simulink model "flexible_joint_v01"  (R2023b)
settings: Solver=FixedStepAuto  StartTime=0.0  StopTime=30  FixedStep=0.001  RelTol=1e-3
settings Model: Creator=GreenTeam  LastModifiedBy=GreenTeam

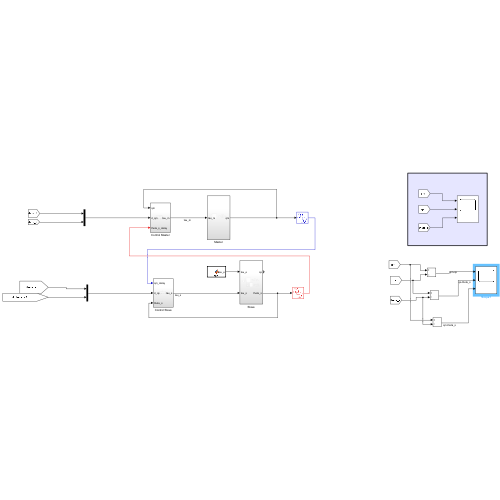
[thumbnail: Simulink's stored preview of the top-level diagram]
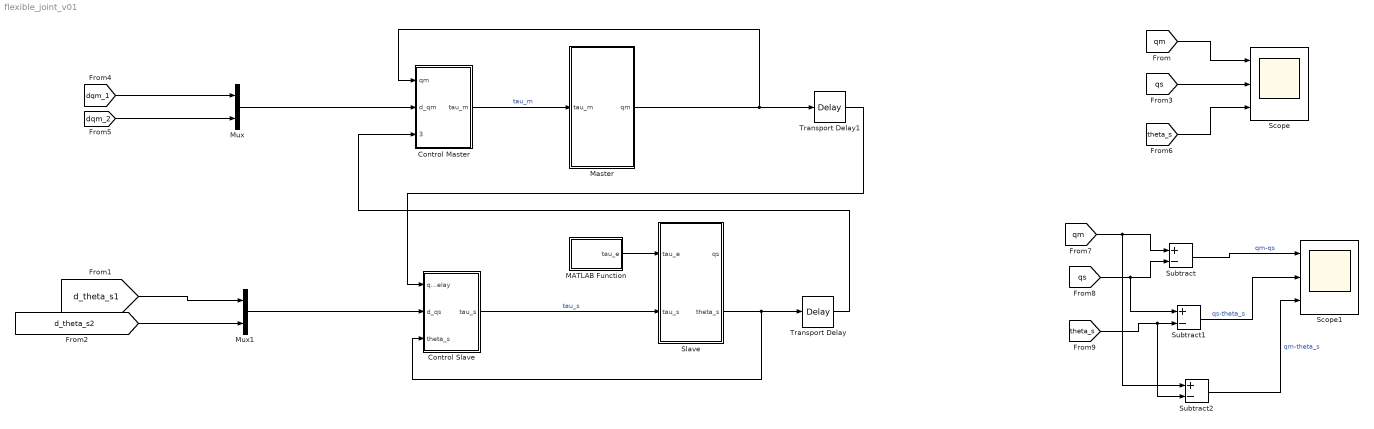
== system flexible_joint_v01 ==
  Control Master : Subsystem
  Control Slave : Subsystem
  MATLAB Function : MATLAB Function  TreatAsAtomicUnit=on
  Master : Subsystem
  Mux : Mux  Inputs=2
  Mux1 : Mux  Inputs=2
  Scope : Scope  NumInputPorts=3
  Scope1 : Scope  NumInputPorts=3
  Slave : Subsystem
  Subtract : Sum  Inputs=+-
  Subtract1 : Sum  Inputs=+-
  Subtract2 : Sum  Inputs=+-
  Transport Delay : TransportDelay  DelayTime=0.55
  Transport Delay1 : TransportDelay  DelayTime=0.55
  wires:
  Control Master/1(tau_m) -> Master/1(tau_m)  "tau_m"
  Slave/2(theta_s) -> Control Slave/3(theta_s), Transport Delay/1
  Control Slave/1(tau_s) -> Slave/2(tau_s)  "tau_s"
  MATLAB Function/1(tau_e) -> Slave/1(tau_e)
  [dqm_2] -> Mux/2
  Mux/1 -> Control Master/2(d_qm)
  [d_theta_s1] -> Mux1/1
  [d_theta_s2] -> Mux1/2
  Mux1/1 -> Control Slave/2(d_qs)
  Master/1(qm) -> Control Master/1(qm), Transport Delay1/1
  Transport Delay/1 -> Control Master/3(theta_s_delay)
  Transport Delay1/1 -> Control Slave/1(qm_delay)
  [dqm_1] -> Mux/1
  [qm] -> Scope/1
  [qs] -> Scope/2
  [theta_s] -> Scope/3
  [qm] -> Subtract2/1, Subtract/1
  [qs] -> Subtract1/1, Subtract/2
  Subtract/1 -> Scope1/1  "qm-qs"
  [theta_s] -> Subtract2/2, Subtract1/2
  Subtract1/1 -> Scope1/2  "qs-theta_s"
  Subtract2/1 -> Scope1/3  "qm-theta_s"

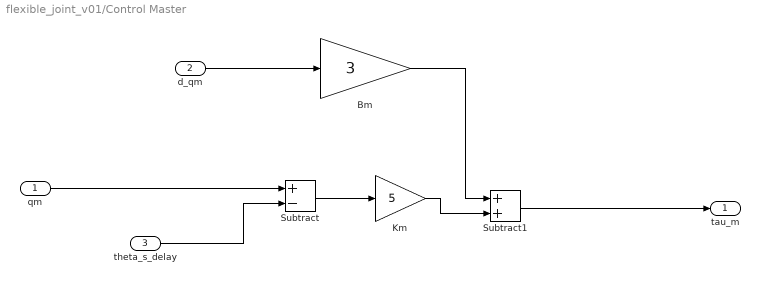
== system flexible_joint_v01/Control Master ==
  qm : Inport
  d_qm : Inport  Port=2
  theta_s_delay : Inport  Port=3
  Bm : Gain  Gain=3
  Km : Gain  Gain=5
  Subtract : Sum  Inputs=+-
  Subtract1 : Sum
  tau_m : Outport
  wires:
  Bm/1 -> Subtract1/1
  Subtract/1 -> Km/1
  Subtract1/1 -> tau_m/1
  Km/1 -> Subtract1/2
  d_qm/1 -> Bm/1
  qm/1 -> Subtract/1
  theta_s_delay/1 -> Subtract/2

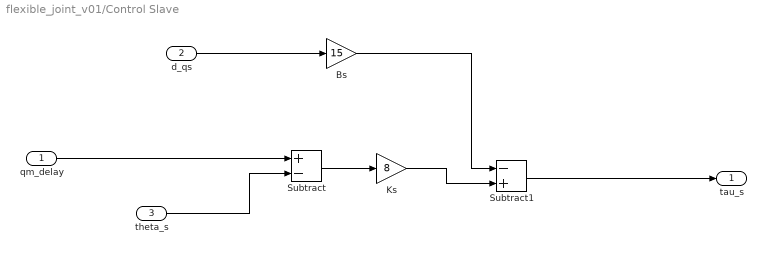
== system flexible_joint_v01/Control Slave ==
  qm_delay : Inport
  d_qs : Inport  Port=2
  theta_s : Inport  Port=3
  Bs : Gain  Gain=15
  Ks : Gain  Gain=8
  Subtract : Sum  Inputs=+-
  Subtract1 : Sum  Inputs=-+
  tau_s : Outport
  wires:
  theta_s/1 -> Subtract/2
  qm_delay/1 -> Subtract/1
  d_qs/1 -> Bs/1
  Ks/1 -> Subtract1/2
  Subtract1/1 -> tau_s/1
  Subtract/1 -> Ks/1
  Bs/1 -> Subtract1/1

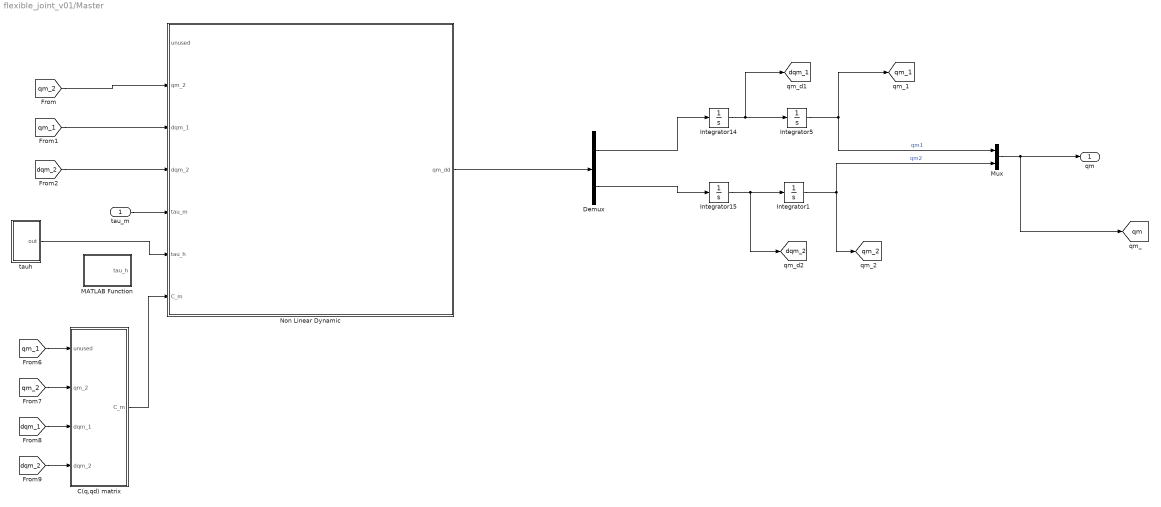
== system flexible_joint_v01/Master ==
  tau_m : Inport
  C(q,qd) matrix : MATLAB Function  TreatAsAtomicUnit=on
  Demux : Demux  Outputs=2
  Integrator1 : Integrator  InitialCondition=1/(8*pi)
  Integrator14 : Integrator
  Integrator15 : Integrator
  Integrator5 : Integrator  InitialCondition=-1/(8*pi)
  MATLAB Function : MATLAB Function  TreatAsAtomicUnit=on
  Mux : Mux  Inputs=2
  Non Linear Dynamic : MATLAB Function  TreatAsAtomicUnit=on
  tauh : Subsystem
  qm : Outport  VectorParamsAs1DForOutWhenUnconnected=off
  tag scope: dqm_1=global, dqm_2=global, qm=global, qm_1=global, qm_2=global
  wires:
  Integrator5/1 -> [qm_1], Mux/1  "qm1"
  Demux/1 -> Integrator14/1
  Non Linear Dynamic/1(qm_dd) -> Demux/1
  Integrator1/1 -> [qm_2], Mux/2  "qm2"
  tau_m/1 -> Non Linear Dynamic/5(tau_m)
  Integrator14/1 -> Integrator5/1, [dqm_1]
  Integrator15/1 -> [dqm_2], Integrator1/1
  Demux/2 -> Integrator15/1
  C(q,qd) matrix/1(C_m) -> Non Linear Dynamic/7(C_m)
  [qm_2] -> Non Linear Dynamic/2(qm_2)
  [dqm_2] -> Non Linear Dynamic/4(dqm_2)
  [qm_1] -> Non Linear Dynamic/3(dqm_1)
  [dqm_1] -> C(q,qd) matrix/3(dqm_1)
  [qm_1] -> C(q,qd) matrix/1(unused)
  [dqm_2] -> C(q,qd) matrix/4(dqm_2)
  [qm_2] -> C(q,qd) matrix/2(qm_2)
  Mux/1 -> [qm], qm/1
  tauh/1(out) -> Non Linear Dynamic/6(tau_h)

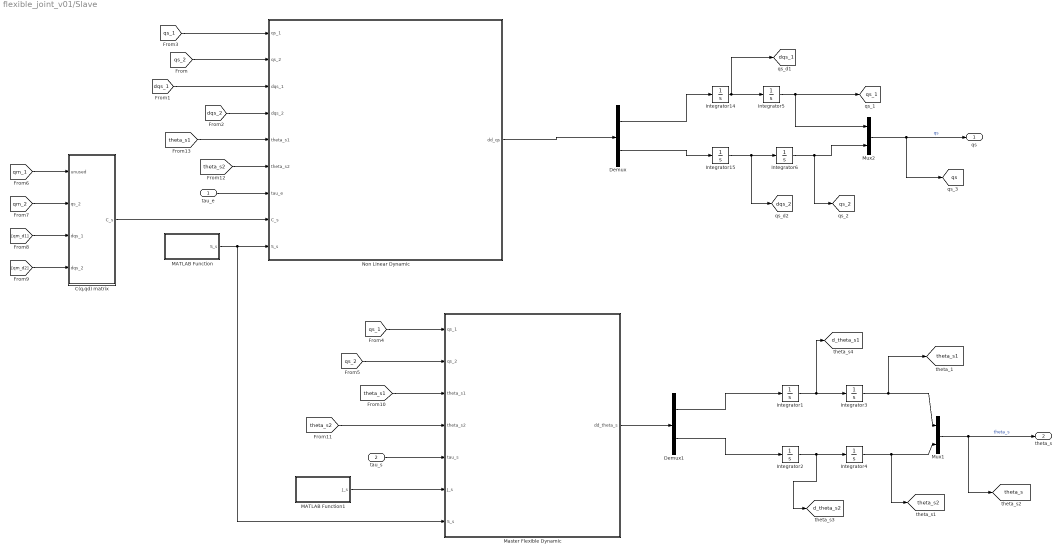
== system flexible_joint_v01/Slave ==
  tau_e : Inport
  tau_s : Inport  Port=2
  C(q,qd) matrix : MATLAB Function  TreatAsAtomicUnit=on
  Demux : Demux  Outputs=2
  Demux1 : Demux  Outputs=2
  Integrator{1..2,14..15} (4 alike) : Integrator
  Integrator3 : Integrator  InitialCondition=1/(5*pi)
  Integrator4 : Integrator  InitialCondition=-1/(2*pi)
  Integrator5 : Integrator  InitialCondition=1/(5*pi)
  Integrator6 : Integrator  InitialCondition=-1/(2*pi)
  MATLAB Function : MATLAB Function  TreatAsAtomicUnit=on
  MATLAB Function1 : MATLAB Function  TreatAsAtomicUnit=on
  Master Flexible Dynamic : MATLAB Function  TreatAsAtomicUnit=on
  Mux1 : Mux  Inputs=2
  Mux2 : Mux  Inputs=2
  Non Linear Dynamic : MATLAB Function  TreatAsAtomicUnit=on
  qs : Outport
  theta_s : Outport  Port=2
  tag scope: d_theta_s1=global, d_theta_s2=global, dqs_1=global, dqs_2=global, qs=global, qs_1=global, qs_2=global, theta_s1=global, theta_s2=global, theta_s=global
  wires:
  [qm_2] -> C(q,qd) matrix/2(qs_2)
  [qm_d2] -> C(q,qd) matrix/4(dqs_2)
  [qm_1] -> C(q,qd) matrix/1(unused)
  [qm_d1] -> C(q,qd) matrix/3(dqs_1)
  [dqs_1] -> Non Linear Dynamic/3(dqs_1)
  [dqs_2] -> Non Linear Dynamic/4(dqs_2)
  [qs_2] -> Non Linear Dynamic/2(qs_2)
  Demux/2 -> Integrator15/1
  Integrator15/1 -> [dqs_2], Integrator6/1
  Integrator14/1 -> [dqs_1], Integrator5/1
  Integrator6/1 -> Mux2/2, [qs_2]
  Non Linear Dynamic/1(dd_qs) -> Demux/1
  Demux/1 -> Integrator14/1
  Mux2/1 -> [qs], qs/1  "qs"
  Integrator5/1 -> [qs_1], Mux2/1
  C(q,qd) matrix/1(C_s) -> Non Linear Dynamic/8(C_s)
  MATLAB Function/1(S_s) -> Non Linear Dynamic/9(S_s), Master Flexible Dynamic/7(S_s)
  [qs_1] -> Non Linear Dynamic/1(qs_1)
  MATLAB Function1/1(J_s) -> Master Flexible Dynamic/6(J_s)
  Integrator3/1 -> [theta_s1], Mux1/1
  Integrator1/1 -> [d_theta_s1], Integrator3/1
  Demux1/1 -> Integrator1/1
  Master Flexible Dynamic/1(dd_theta_s) -> Demux1/1
  Integrator4/1 -> Mux1/2, [theta_s2]
  Integrator2/1 -> [d_theta_s2], Integrator4/1
  Mux1/1 -> [theta_s], theta_s/1  "theta_s"
  Demux1/2 -> Integrator2/1
  [qs_1] -> Master Flexible Dynamic/1(qs_1)
  [qs_2] -> Master Flexible Dynamic/2(qs_2)
  [theta_s1] -> Master Flexible Dynamic/3(theta_s1)
  [theta_s2] -> Master Flexible Dynamic/4(theta_s2)
  [theta_s2] -> Non Linear Dynamic/6(theta_s2)
  [theta_s1] -> Non Linear Dynamic/5(theta_s1)
  tau_e/1 -> Non Linear Dynamic/7(tau_e)
  tau_s/1 -> Master Flexible Dynamic/5(tau_s)

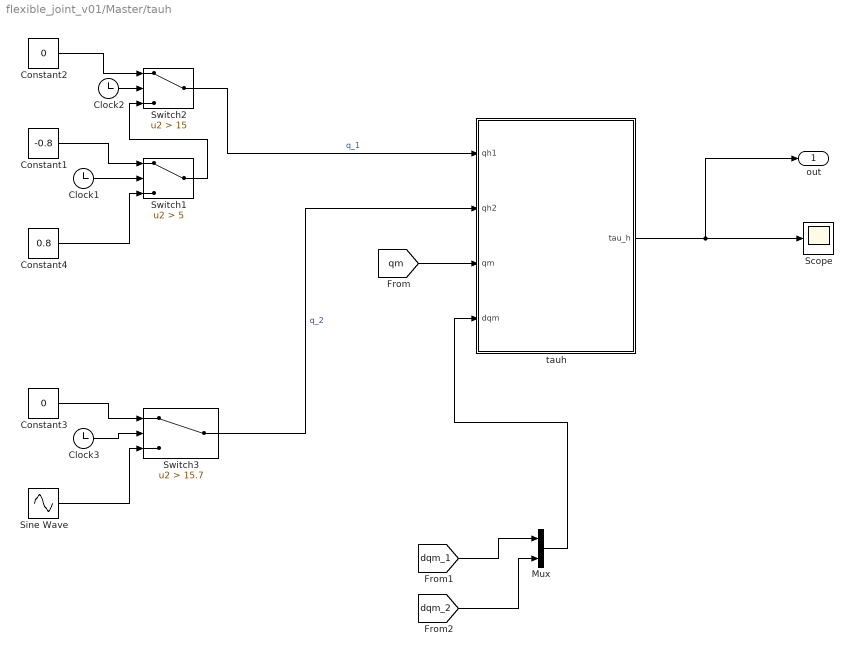
== system flexible_joint_v01/Master/tauh ==
  Clock1 : Clock
  Clock2 : Clock
  Clock3 : Clock
  Constant1 : Constant  Value=-0.8
  Constant2 : Constant  Value=0
  Constant3 : Constant  Value=0
  Constant4 : Constant  Value=0.8
  Mux : Mux  Inputs=2
  Scope : Scope
  Sine Wave : Sin  Amplitude=1.5  Frequency=0.2  SampleTime=0
  Switch1 : Switch  Criteria=u2 > Threshold  Threshold=5  SaturateOnIntegerOverflow=off  InputSameDT=off
  Switch2 : Switch  Criteria=u2 > Threshold  Threshold=15  SaturateOnIntegerOverflow=off  InputSameDT=off
  Switch3 : Switch  Criteria=u2 > Threshold  Threshold=15.7  SaturateOnIntegerOverflow=off  InputSameDT=off
  tauh : MATLAB Function  TreatAsAtomicUnit=on
  out : Outport
  wires:
  tauh/1(tau_h) -> out/1, Scope/1
  Switch3/1 -> tauh/2(qh2)  "q_2"
  Switch2/1 -> tauh/1(qh1)  "q_1"
  Sine Wave/1 -> Switch3/3
  Clock3/1 -> Switch3/2
  Constant3/1 -> Switch3/1
  Constant1/1 -> Switch1/1
  Constant2/1 -> Switch2/1
  Clock2/1 -> Switch2/2
  Switch1/1 -> Switch2/3
  Clock1/1 -> Switch1/2
  Constant4/1 -> Switch1/3
  [dqm_1] -> Mux/1
  [dqm_2] -> Mux/2
  Mux/1 -> tauh/4(dqm)
  [qm] -> tauh/3(qm)

== matlab function flexible_joint_v01/Master/tauh/tauh ==
  data: qh1 input; qh2 input; qm input; tau_h output; dqm input
function tau_h = spring_damper(qh1,qh2,qm,dqm)

Kh=10;
Dh=2;

qh=[qh1;qh2];
tau_h=Kh*(qh-qm)-Dh*dqm;


end

== matlab function flexible_joint_v01/Master/C(q,qd) matrix ==
  data: unused input; qm_2 input; dqm_1 input; C_m output; dqm_2 input
function C_m = fcn(~,qm_2,dqm_1,dqm_2)

% Phyiscal Parameters
Lm1 = 0.38;                                          %Master_first_link_length
Lm2 = 0.38;                                          %Master_second_link_length
mm1 = 3.5;                                           %Master_first_link_mass
mm2 = 0.5;                                           %Master_second_link_mass

betha_m=Lm1*Lm2*mm2;

C_m_11 = -2*betha_m*sin(qm_2)*dqm_2;
C_m_12 = -betha_m*sin(qm_2)*dqm_2;
C_m_21 =  betha_m*sin(qm_2)*dqm_1;
C_m_22 =  0;
C_m = [C_m_11 C_m_12; C_m_21 C_m_22];
end

== matlab function flexible_joint_v01/Master/Non Linear Dynamic ==
  data: unused input; qm_2 input; dqm_1 input; dqm_2 input; tau_m input; tau_h input; qm_dd output; C_m input
function qm_dd =fcn(~,qm_2,dqm_1,dqm_2,tau_m,tau_h,C_m)

% Phyiscal Parameters
Lm1 = 0.38;                                          %Master_first_link_length
Lm2 = 0.38;                                          %Master_second_link_length
mm1 = 3.5;                                           %Master_first_link_mass
mm2 = 0.5;                                           %Master_second_link_mass

dqm=[dqm_1;dqm_2];
alpha_m=(Lm2^2)*mm2+(Lm1^2)*(mm1+mm2);
betha_m=Lm1*Lm2*mm2;
delta_m=(Lm2^2)*mm2;

M_m_11= alpha_m + 2*betha_m*cos(qm_2);  
M_m_12= delta_m + betha_m * cos(qm_2);
M_m_21= M_m_12;
M_m_22= delta_m;
M_m = [M_m_11 M_m_12; M_m_21 M_m_22];
qm_dd = inv(M_m)*( -tau_m -(C_m * dqm ) + tau_h );
end

== matlab function flexible_joint_v01/Slave/C(q,qd) matrix ==
  data: unused input; qs_2 input; dqs_1 input; C_s output; dqs_2 input
function C_s = fcn(~,qs_2,dqs_1,dqs_2)

% Phyiscal Parameters
Ls1 = 0.38;                                          %Slave_first_link_length
Ls2 = 0.38;                                          %Slave_second_link_length
ms1 = 0.5;                                           %Slave_first_link_mass
ms2 = 0.35;                                          %Slave_second_link_mass

betha_s=Ls1*Ls2*ms2;

C_s_11 = -2*betha_s*sin(qs_2)*dqs_2;
C_s_12 = -betha_s*sin(qs_2)*dqs_2;
C_s_21 =  betha_s*sin(qs_2)*dqs_1;
C_s_22 =  0;
C_s= [C_s_11 C_s_12; C_s_21 C_s_22];
end

== matlab function flexible_joint_v01/Slave/Non Linear Dynamic ==
  data: qs_1 input; qs_2 input; dqs_1 input; dqs_2 input; theta_s1 input; theta_s2 input; dd_qs output; tau_e input; C_s input; S_s input
function dd_qs =Rigid_Body_Slave(qs_1,qs_2,dqs_1,dqs_2,theta_s1,theta_s2,tau_e,C_s,S_s)

% Phyiscal Parameters
Ls1 = 0.38;                                          %Slave_first_link_length
Ls2 = 0.38;                                          %Slave_second_link_length
ms1 = 0.5;                                           %Slave_first_link_mass
ms2 = 0.35;                                          %Slave_second_link_mass

qs=[qs_1;qs_2];
theta_s=[theta_s1;theta_s2];
dqs=[dqs_1;dqs_2];
alpha_s=(Ls2^2)*ms2+(Ls1^2)*(ms1+ms2);
betha_s=Ls1*Ls2*ms2;
delta_s=(Ls2^2)*ms2;

M_s_11= alpha_s + 2*betha_s*cos(qs_2);  
M_s_12= delta_s + betha_s * cos(qs_2);
M_s_21= M_s_12;
M_s_22= delta_s;
M_s = [M_s_11 M_s_12; M_s_21 M_s_22];
dd_qs= inv(M_s)*(- tau_e  - (C_s * dqs ) - (S_s*(qs-theta_s)));
end

== matlab function flexible_joint_v01/Slave/MATLAB Function ==
  data: S_s output
function S_s = Stifness_Matrix()
    % This function creates a 2x2 identity matrix scaled by 500

    % Create a 2x2 identity matrix
    I = eye(2);
    
    % Scale the identity matrix by 500
    S_s = 500 * I;
end

== matlab function flexible_joint_v01/Slave/Master Flexible Dynamic ==
  data: qs_1 input; qs_2 input; theta_s1 input; dd_theta_s output; theta_s2 input; tau_s input; J_s input; S_s input
function dd_theta_s = Flex_Body_Slave(qs_1,qs_2,theta_s1,theta_s2,tau_s,J_s,S_s)

qs=[qs_1;qs_2];
theta_s=[theta_s1;theta_s2];


dd_theta_s = inv(J_s)*(tau_s - S_s*(theta_s-qs));

end

== matlab function flexible_joint_v01/Slave/MATLAB Function1 ==
  data: J_s output
function J_s = Inertia_Matrix()

    % Create a 2x2 identity matrix
    I = eye(2);
    % Scale the identity matrix by 500
    J_s = 0.2 * I;
end

== matlab function flexible_joint_v01/MATLAB Function ==
  data: tau_e output
function tau_e = fcn()

tau_e=[0;0];

== matlab function flexible_joint_v01/Master/MATLAB Function ==
  data: tau_h output
function tau_h = fcn()

tau_h=[0;0];
